simulink model "sim1"  (R2024a)
settings: Solver=FixedStepAuto  StartTime=0.0  StopTime=5.0  FixedStep=1e-3  RelTol=1e-3
InitFcn:
  | A=[0 1;
  |     -2 4];
  | b=[8;
  |     9];
  | Q=[3 0;
  |     0 4];
  | r=4;
  | K=[-6.310,7.594];
libraries: matrix_library x1
settings Model: Creator=alexe  LastModifiedBy=alexe

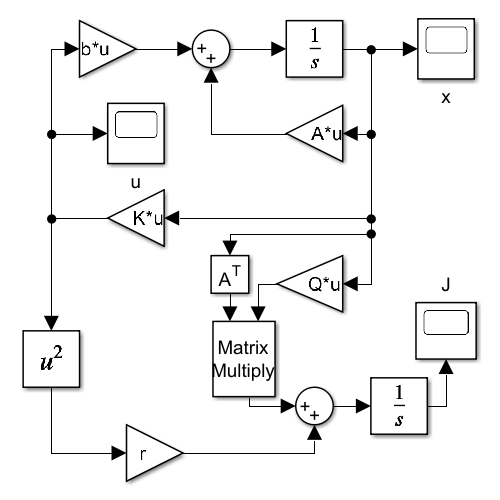
[thumbnail: Simulink's stored preview of the top-level diagram]
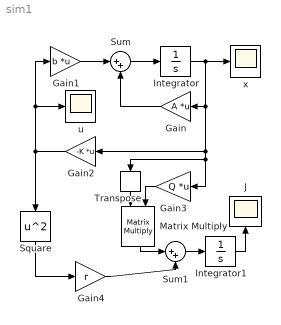
== system sim1 ==
  Gain : Gain  Gain=A  Multiplication=Matrix(K*u)
  Gain1 : Gain  Gain=b  Multiplication=Matrix(K*u)
  Gain2 : Gain  Gain=-K  Multiplication=Matrix(K*u)
  Gain3 : Gain  Gain=Q  Multiplication=Matrix(K*u)
  Gain4 : Gain  Gain=r
  Integrator : Integrator  InitialCondition=[1;0]
  Integrator1 : Integrator
  J : Scope
  Matrix Multiply : Product  Multiplication=Matrix(*)
  Square : Math  Operator=square
  Sum : Sum  Inputs=|++
  Sum1 : Sum  Inputs=|++
  Transpose : matrix_library/Transpose
  u : Scope
  x : Scope
  wires:
  Integrator/1 -> x/1, Gain3/1, Transpose/1, Gain2/1, Gain/1
  Gain/1 -> Sum/2
  Gain1/1 -> Sum/1
  Sum/1 -> Integrator/1
  Gain2/1 -> Square/1, u/1, Gain1/1
  Matrix Multiply/1 -> Sum1/1
  Square/1 -> Gain4/1
  Gain4/1 -> Sum1/2
  Sum1/1 -> Integrator1/1
  Integrator1/1 -> J/1
  Gain3/1 -> Matrix Multiply/2
  Transpose/1 -> Matrix Multiply/1
